simulink subsystem "FirstHouse"  (R2023a)
settings: Solver=VariableStepAuto  StartTime=0.0  StopTime=10.0  RelTol=1e-3
undefined symbols (not defined in the file): A, K
libraries: mpclib x1
settings Model: Creator=giaco  LastModifiedBy=giaco

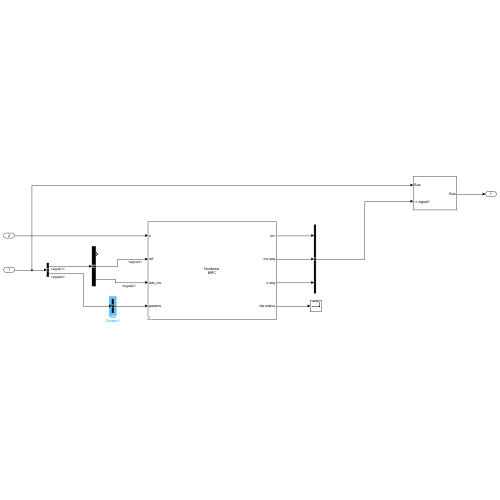
[thumbnail: Simulink's stored preview of the top-level diagram]
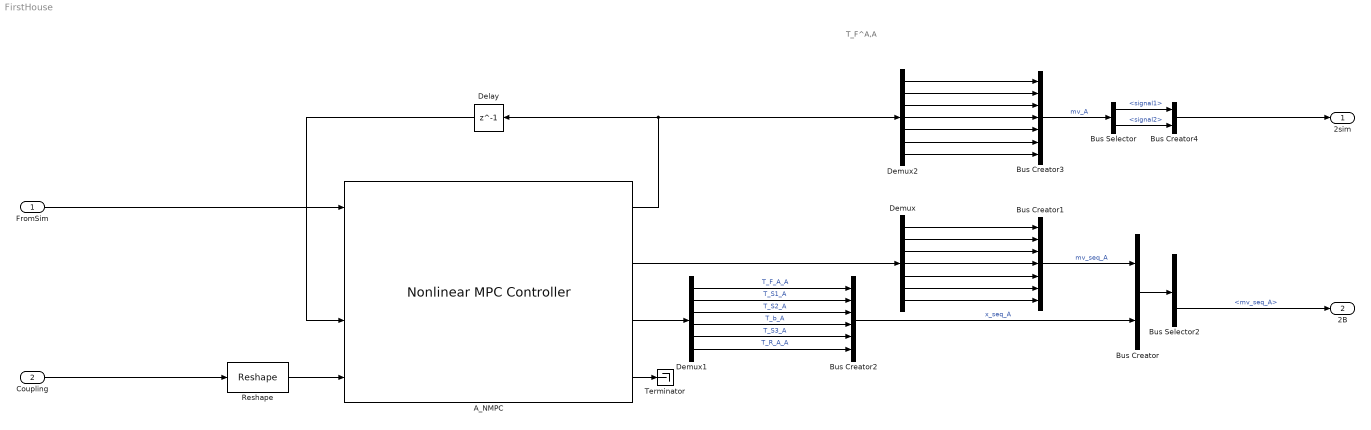
== system FirstHouse ==
  note: T_F^A,A
  FromSim : Inport
  Coupling : Inport  Port=2
  A_NMPC : mpclib/Nonlinear MPC Controller  UseObjectTs=on  UseMEX=off  md_enabled=on  mvtarget_enabled=off  param_enabled=off  cost_enabled=off  mvseq_enabled=on  stateseq_enabled=on  ovseq_enabled=off  slack_enabled=off  status_enabled=on  ov_min=off  ov_max=off  mv_min=off  mv_max=off  mvrate_min=off  mvrate_max=off  state_min=off  state_max=off  ov_weight=off  mv_weight=off  mvrate_weight=off  ecr_weight=off  nlp_initialize=off
  Bus Creator : BusCreator  Inputs=2
  Bus Creator1 : BusCreator  Inputs=7
  Bus Creator2 : BusCreator  Inputs=6
  Bus Creator3 : BusCreator  Inputs=7
  Bus Creator4 : BusCreator  Inputs=2
  Bus Selector : BusSelector  OutputSignals=signal1,signal2
  Bus Selector2 : BusSelector  OutputSignals=signal1,mv_seq_A
  Delay : Delay  DelayLength=1
  Demux : Demux  Outputs=7
  Demux1 : Demux  Outputs=6
  Demux2 : Demux  Outputs=7
  Reshape : Reshape  OutputDimensionality=Customize  OutputDimensions=[K,A.nu_md]
  Terminator : Terminator
  2sim : Outport
  2B : Outport  Port=2
  wires:
  A_NMPC/4 -> Terminator/1
  A_NMPC/2 -> Demux/1
  A_NMPC/3 -> Demux1/1
  Delay/1 -> A_NMPC/3
  FromSim/1 -> A_NMPC/1
  Reshape/1 -> A_NMPC/4
  Coupling/1 -> Reshape/1
  Bus Creator/1 -> Bus Selector2/1
  Bus Selector2/2 -> 2B/1  "<mv_seq_A>"
  Demux/1 -> Bus Creator1/1
  Demux/2 -> Bus Creator1/2
  Demux/3 -> Bus Creator1/3
  Demux/4 -> Bus Creator1/4
  Demux/5 -> Bus Creator1/5
  Demux/6 -> Bus Creator1/6
  Demux/7 -> Bus Creator1/7
  Bus Creator1/1 -> Bus Creator/1  "mv_seq_A"
  Demux1/6 -> Bus Creator2/6  "T_R_A_A"
  Demux1/5 -> Bus Creator2/5  "T_S3_A"
  Demux1/4 -> Bus Creator2/4  "T_b_A"
  Demux1/3 -> Bus Creator2/3  "T_S2_A"
  Demux1/2 -> Bus Creator2/2  "T_S1_A"
  Demux1/1 -> Bus Creator2/1  "T_F_A_A"
  Bus Creator2/1 -> Bus Creator/2  "x_seq_A"
  Demux2/1 -> Bus Creator3/1
  A_NMPC/1 -> Delay/1, Demux2/1
  Demux2/4 -> Bus Creator3/4
  Bus Creator3/1 -> Bus Selector/1  "mv_A"
  Demux2/6 -> Bus Creator3/6
  Demux2/2 -> Bus Creator3/2
  Demux2/7 -> Bus Creator3/7
  Demux2/3 -> Bus Creator3/3
  Demux2/5 -> Bus Creator3/5
  Bus Selector/1 -> Bus Creator4/1  "<signal1>"
  Bus Selector/2 -> Bus Creator4/2  "<signal2>"
  Bus Creator4/1 -> 2sim/1
